simulink model "Cap2_Ex2"  (R2022b)
settings: Solver=VariableStepAuto  StartTime=0.0  StopTime=10.0  RelTol=1e-3
values from neighbouring files (symbols this model uses):
  b = 5000    [Cap2_Ex2_script.m]
  k1 = 120000    [Cap2_Ex2_script.m]
  k2 = 100    [Cap2_Ex2_script.m]
  m1 = 20    [Cap2_Ex2_script.m]
  m2 = 100    [Cap2_Ex2_script.m]
settings Model: Creator=Pedro Lamego  LastModifiedBy=Gonçalo Bastos
settings DataIOCC: Refine=1000
settings DebuggingCC: UnconnectedInputMsg=warning  UnconnectedOutputMsg=warning  UnconnectedLineMsg=warning
settings ModelReferenceCC: EnableRefExpFcnMdlSchedulingChecks=on
settings RTWCC: DLArmComputeVersion=19.05

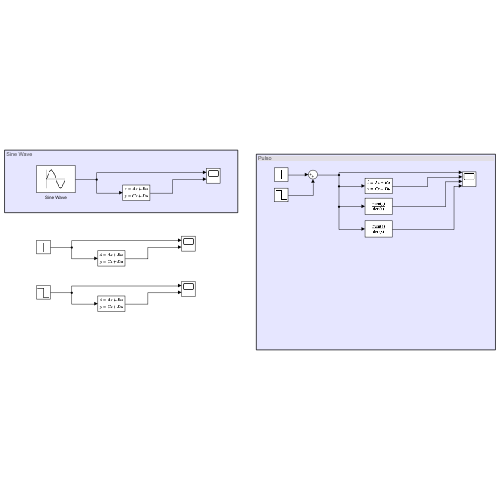
[thumbnail: Simulink's stored preview of the top-level diagram]
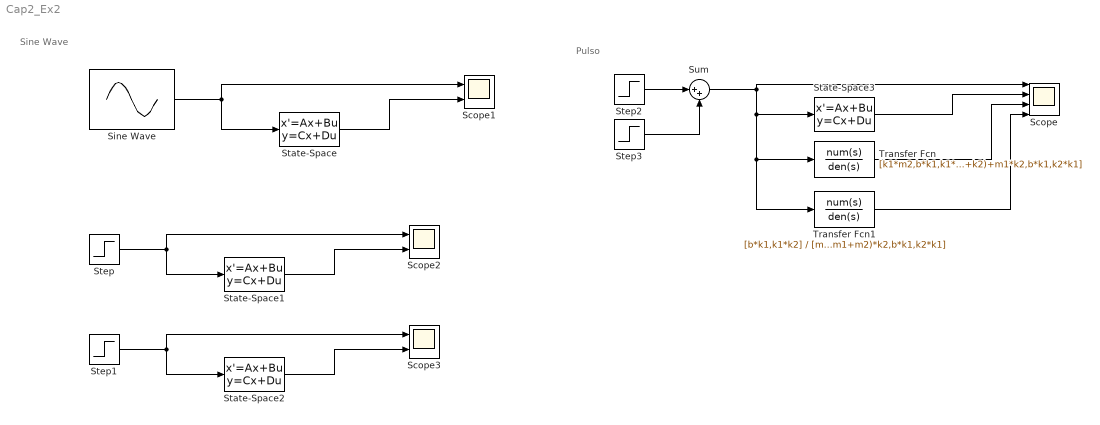
== system Cap2_Ex2 ==
  note: Pulso
  note: Sine Wave
  Scope : Scope  NumInputPorts=4
  Scope1 : Scope  NumInputPorts=2
  Scope2 : Scope  NumInputPorts=2
  Scope3 : Scope  NumInputPorts=2
  Sine Wave : Sin  SampleTime=0
  State-Space{,1..3} (4 alike) : StateSpace  A=[0 0 1 0; 0 0 0 1; -(k1+k2)/m1 k2/m1 -b/m1 b/m1; k2/m2 -k2/m2 b/m2 -b/m2]  B=[0; 0; k1/m1; 0]  C=[1 0 0 0; 0 1 0 0]  D=[0;0]  InitialCondition=0
  Step : Step  SampleTime=0
  Step1 : Step  Before=1  After=0  SampleTime=0
  Step2 : Step  After=0.2  SampleTime=0  ZeroCross=off
  Step3 : Step  Time=0.25  After=-0.2  SampleTime=0
  Sum : Sum  Inputs=|++
  Transfer Fcn : TransferFcn  Numerator=[k1*m2,b*k1,k1*k2]  Denominator=[m1*m2, b*(m1+m2),m2*(k1+k2)+m1*k2,b*k1,k2*k1]
  Transfer Fcn1 : TransferFcn  Numerator=[b*k1,k1*k2]  Denominator=[m1*m2, b*(m1+m2),k1*m2+(m1+m2)*k2,b*k1,k2*k1]
  wires:
  Transfer Fcn1/1 -> Scope/4
  State-Space3/1 -> Scope/2
  Step/1 -> State-Space1/1, Scope2/1
  State-Space2/1 -> Scope3/2
  State-Space/1 -> Scope1/2
  Step3/1 -> Sum/2
  Sine Wave/1 -> State-Space/1, Scope1/1
  Step2/1 -> Sum/1
  Step1/1 -> State-Space2/1, Scope3/1
  Sum/1 -> Scope/1, State-Space3/1, Transfer Fcn1/1, Transfer Fcn/1
  Transfer Fcn/1 -> Scope/3
  State-Space1/1 -> Scope2/2
